simulink model "Simulazione_Moto"  (R2020b)
settings: Solver=VariableStepAuto  StartTime=0.0  StopTime=10  RelTol=1e-3
InitFcn:
  | Inizializzazione
StopFcn:
  | visualizzazione
values from neighbouring files (symbols this model uses):
  R0 = [x0; y0; th0]    [Inizializzazione.m]
  R0r = [x0r; y0r; th0r]    [Inizializzazione.m]
settings Model: Creator=andre  LastModifiedBy=andre

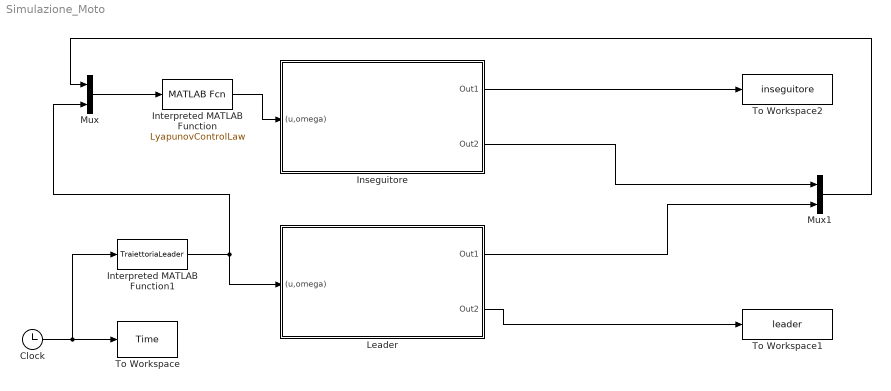
== system Simulazione_Moto ==
  Clock : Clock
  Inseguitore : Subsystem
  Interpreted MATLAB Function : MATLABFcn  MATLABFcn=LyapunovControlLaw
  Interpreted MATLAB Function1 : MATLABFcn  MATLABFcn=TraiettoriaLeader  OutputDimensions=2
  Leader : Subsystem
  Mux : Mux  Inputs=2
  Mux1 : Mux  Inputs=2
  To Workspace : ToWorkspace  VariableName=Time  SaveFormat=Timeseries  SampleTime=-1
  To Workspace1 : ToWorkspace  VariableName=leader  SampleTime=-1
  To Workspace2 : ToWorkspace  VariableName=inseguitore  SampleTime=-1
  wires:
  Interpreted MATLAB Function/1 -> Inseguitore/1((u,omega))
  Mux/1 -> Interpreted MATLAB Function/1
  Mux1/1 -> Mux/1
  Leader/1(Out1) -> Mux1/2
  Interpreted MATLAB Function1/1 -> Leader/1((u,omega)), Mux/2
  Clock/1 -> Interpreted MATLAB Function1/1, To Workspace/1
  Inseguitore/2(Out2) -> Mux1/1
  Inseguitore/1(Out1) -> To Workspace2/1
  Leader/2(Out2) -> To Workspace1/1

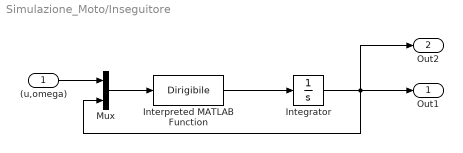
== system Simulazione_Moto/Inseguitore ==
  (u,omega) : Inport
  Integrator : Integrator  InitialCondition=R0
  Interpreted MATLAB Function : MATLABFcn  MATLABFcn=Dirigibile
  Mux : Mux  Inputs=2
  Out1 : Outport
  Out2 : Outport  Port=2
  wires:
  Interpreted MATLAB Function/1 -> Integrator/1
  Integrator/1 -> Mux/2, Out2/1, Out1/1
  Mux/1 -> Interpreted MATLAB Function/1
  (u,omega)/1 -> Mux/1

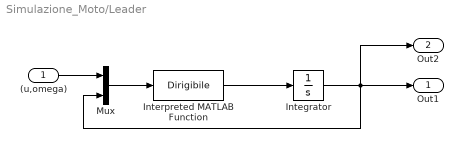
== system Simulazione_Moto/Leader ==
  (u,omega) : Inport
  Integrator : Integrator  InitialCondition=R0r
  Interpreted MATLAB Function : MATLABFcn  MATLABFcn=Dirigibile
  Mux : Mux  Inputs=2
  Out1 : Outport
  Out2 : Outport  Port=2
  wires:
  Interpreted MATLAB Function/1 -> Integrator/1
  Integrator/1 -> Mux/2, Out2/1, Out1/1
  Mux/1 -> Interpreted MATLAB Function/1
  (u,omega)/1 -> Mux/1
